simulink model "vcm"  (R2024b)
settings: Solver=VariableStepAuto  StartTime=0.0  StopTime=0.03  RelTol=1e-3
values from neighbouring files (symbols this model uses):
  Da = 0    [one_axis_servo.m]
  Ja = 0.00196    [one_axis_servo.m]
  KT = 0.912    [one_axis_servo.m]
  Kvi = Wvc/5    (= 100)    [one_axis_servo.m]
  Kvp = Ja*Wvc/KT    (= 1.07456140351)    [one_axis_servo.m]
  vfb_on = 1    [one_axis_servo.m]
  Wcc = 5*Wvc    (= 2500)    [one_axis_servo.m]
undefined symbols (not defined in the file or in its folder): Tdv
settings Model: Creator=shohei  LastModifiedBy=shohei

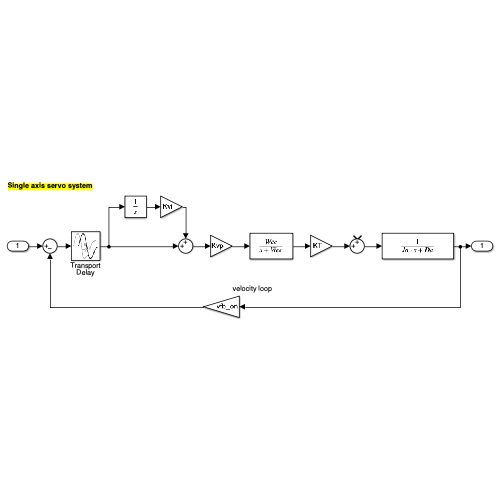
[thumbnail: Simulink's stored preview of the top-level diagram]
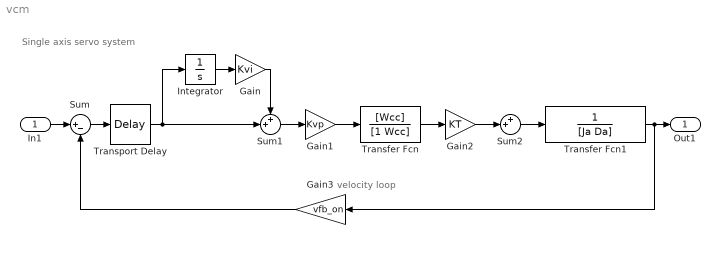
== system vcm ==
  note: Single axis servo system
  note: velocity loop
  In1 : Inport
  Gain : Gain  Gain=Kvi
  Gain1 : Gain  Gain=Kvp
  Gain2 : Gain  Gain=KT
  Gain3 : Gain  Gain=vfb_on
  Integrator : Integrator
  Sum : Sum  Inputs=|+-
  Sum1 : Sum  Inputs=++|
  Sum2 : Sum  Inputs=++|
  Transfer Fcn : TransferFcn  Numerator=[Wcc]  Denominator=[1 Wcc]
  Transfer Fcn1 : TransferFcn  Denominator=[Ja Da]
  Transport Delay : TransportDelay  DelayTime=Tdv  PadeOrder=n
  Out1 : Outport
  wires:
  In1/1 -> Sum/1
  Integrator/1 -> Gain/1
  Gain/1 -> Sum1/1
  Sum1/1 -> Gain1/1
  Gain1/1 -> Transfer Fcn/1
  Transfer Fcn/1 -> Gain2/1
  Gain2/1 -> Sum2/2
  Sum2/1 -> Transfer Fcn1/1
  Transfer Fcn1/1 -> Gain3/1, Out1/1
  Gain3/1 -> Sum/2
  Sum/1 -> Transport Delay/1
  Transport Delay/1 -> Integrator/1, Sum1/2
